simulink model "benchmark_ivan_PIANN"  (R2024b)
settings: Solver=FixedStepAuto  StartTime=0.0  StopTime=14  FixedStep=0.0001  RelTol=1e-5  AbsTol=1e-8  EnableMultiTasking=on
values from neighbouring files (symbols this model uses):
  b1 = csvread('./DAE_ANN/ANN/Biases/30_04_21/lstm_ann_pi_standard_fix_noSo4_rnn_1__100_16_b_3.csv')    [init_PI_ann.m]    (also in init_PI_ann_hier.m = csvread('./DAE_ANN/ANN/Biases/12_05_21/lstm_ann_pi_standard_; init_PI_ann_hier_v2.m = csvread('./DAE_ANN/ANN/Biases/12_05_21/lstm_ann_pi_standard_; init_PI_ann_lab.m = csvread('./DAE_ANN/ANN/Biases/12_05_21/lstm_ann_pi_standard_)
  b2 = csvread('./DAE_ANN/ANN/Biases/30_04_21/lstm_ann_pi_standard_fix_noSo4_rnn_1__100_16_b_3.csv')    [init_PI_ann.m]    (also in init_PI_ann_hier.m = csvread('./DAE_ANN/ANN/Biases/12_05_21/lstm_ann_pi_standard_; init_PI_ann_hier_v2.m = csvread('./DAE_ANN/ANN/Biases/12_05_21/lstm_ann_pi_standard_; init_PI_ann_lab.m = csvread('./DAE_ANN/ANN/Biases/12_05_21/lstm_ann_pi_standard_)
  b_last = csvread('./DAE_ANN/ANN/Biases/12_05_21/lstm_ann_pi_standard_fix_noSo4_last__100_1_b_2.csv')'    [init_PI_ann_hier.m]    (also in init_PI_ann_hier_v2.m; init_PI_ann_lab.m)
  b_out = csvread('./DAE_ANN/ANN/Biases/30_04_21/lstm_ann_pi_standard_fix_noSo4_final__100_16_b_3.csv')    [init_PI_ann.m]    (also in init_PI_ann_hier.m = csvread('./DAE_ANN/ANN/Biases/12_05_21/lstm_ann_pi_standard_; init_PI_ann_hier_v2.m = csvread('./DAE_ANN/ANN/Biases/12_05_21/lstm_ann_pi_standard_; init_PI_ann_lab.m = csvread('./DAE_ANN/ANN/Biases/12_05_21/lstm_ann_pi_standard_)
  ic_sw_Kla = 145*ones(n_sw,1)    [init_PI_ann.m]    (also in init_PI_ann_hier.m; init_PI_ann_hier_v2.m; init_PI_ann_lab.m)
  ic_sw_Snh4 = 6*ones(n_sw,1)    [init_PI_ann.m]    (also in init_PI_ann_hier.m; init_PI_ann_hier_v2.m; init_PI_ann_lab.m)
  ic_sw_Sno4 = 8*ones(n_sw,1)    [init_PI_ann.m]    (also in init_PI_ann_hier.m; init_PI_ann_hier_v2.m; init_PI_ann_lab.m)
  ic_sw_So4 = 3*ones(n_sw,1)    [init_PI_ann.m]    (also in init_PI_ann_hier.m; init_PI_ann_hier_v2.m; init_PI_ann_lab.m)
  ic_sw_So5 = 2*ones(n_sw,1)    [init_PI_ann.m]    (also in init_PI_ann_hier.m; init_PI_ann_hier_v2.m; init_PI_ann_lab.m)
  KLa5_max = 360    [sensorinit.m]
  max_Q4 = 100000    [sensorinit.m]
  max_SNH4 = 20    [sensorinit.m]
  max_SNO2 = 20    [sensorinit.m]
  max_SNO4 = 20    [sensorinit.m]
  max_SO4 = 10    [sensorinit.m]
  max_SO5 = 10    [sensorinit.m]    (also in setup_Prac5.m = 5)
  max_TSS4 = 10000    [sensorinit.m]
  mean_scaler_dir = csvread('./DAE_ANN/ANN/Scalers/30_04_21_lstm_ann_pi_standard_fix_noSo4/mean_scaler_lstm_ann_pi_standard_fix_noSo4.csv')    [init_PI_ann.m]    (also in init_PI_ann_hier.m = csvread('./DAE_ANN/ANN/Scalers/12_05_21_lstm_ann_pi_standard; init_PI_ann_hier_v2.m = csvread('./DAE_ANN/ANN/Scalers/12_05_21_lstm_ann_pi_standard; setup_Prac5.m = [(Q/k)^2, 1.9756, 0.0000, 0]')
  mean_scaler_dir_out = csvread('./DAE_ANN/ANN/Scalers/30_04_21_lstm_ann_pi_standard_fix_noSo4/mean_scaler_lstm_ann_pi_standard_fix_noSo4_out.csv')    [init_PI_ann.m]    (also in init_PI_ann_hier.m = csvread('./DAE_ANN/ANN/Scalers/12_05_21_lstm_ann_pi_standard; init_PI_ann_hier_v2.m = csvread('./DAE_ANN/ANN/Scalers/12_05_21_lstm_ann_pi_standard; setup_Prac5.m = 0)
  min_Q4 = 0    [sensorinit.m]
  min_SNH4 = 0    [sensorinit.m]
  min_SNO2 = 0    [sensorinit.m]
  min_SNO4 = 0    [sensorinit.m]
  min_SO5 = 0    [sensorinit.m]
  min_TSS4 = 0    [sensorinit.m]
  n_layers = 1    [init_PI_ann.m]    (also in init_PI_ann_hier.m; init_PI_ann_hier_v2.m; init_PI_ann_lab.m)
  n_sw = 16    [init_PI_ann.m]    (also in init_PI_ann_hier.m = 1; init_PI_ann_hier_v2.m = 1; init_PI_ann_lab.m = 1)
  n_sw_inverse = 16    [init_PI_ann.m]    (also in init_PI_ann_hier.m = 1; init_PI_ann_hier_v2.m = 1; init_PI_ann_lab.m = 1)
  noiseseed_Q4 = 1    [sensorinit.m]
  noiseseed_SNH4 = 2    [sensorinit.m]
  noiseseed_SNO2 = 2    [sensorinit.m]
  noiseseed_SNO4 = 2    [sensorinit.m]
  noiseseed_SO4 = 2    [sensorinit.m]
  noiseseed_SO5 = 1    [sensorinit.m]
  noiseseed_TSS4 = 1    [sensorinit.m]
  noisesource_Q4 = 1    [sensorinit.m]
  noisesource_SNH4 = 1    [sensorinit.m]
  noisesource_SNO2 = 1    [sensorinit.m]
  noisesource_SNO4 = 1    [sensorinit.m]
  noisesource_SO4 = 1    [sensorinit.m]
  noisesource_SO5 = 1    [sensorinit.m]
  noisesource_TSS4 = 1    [sensorinit.m]
  Qin0 = 18446    [states.mat]
  Qintr = 12141.8126939    [states.mat]
  Qintr_max = 5*Qin0    [sensorinit.m]
  Qintrawstate = 114243.527362    [states.mat]
  Qintrintstate = -116205.765277    [states.mat]
  SETTLERINIT = [12.5979803087 18.2981709885 29.6744598765 68.7829340492 352.293497132 353.981663079 351.499035887 351.323930185 355.679725774 6417.21684783 30 30 ... (80 elements, 1x80)]    [states.mat]
  Sno_mean = 1    [run_bsm1_PIANN_variable.m]
  SO5awstate = 469.399689831    [states.mat]
  SO5intstate = -450.70071346    [states.mat]
  SO5ref = 2    [run_bsm1_PIANN.m]    (also in run_bsm1_PIANN_variable.m)
  So_mean = 2    [run_bsm1_PIANN_variable.m]    (also in setup_Prac5.m = 0.2)
  std_Q4 = 0.025    [sensorinit.m]
  std_scaler_dir = csvread('./DAE_ANN/ANN/Scalers/30_04_21_lstm_ann_pi_standard_fix_noSo4/std_scaler_lstm_ann_pi_standard_fix_noSo4.csv')    [init_PI_ann.m]    (also in init_PI_ann_hier.m = csvread('./DAE_ANN/ANN/Scalers/12_05_21_lstm_ann_pi_standard; init_PI_ann_hier_v2.m = csvread('./DAE_ANN/ANN/Scalers/12_05_21_lstm_ann_pi_standard; setup_Prac5.m = [1, 0.7579, 0.05, 1]')
  std_scaler_dir_out = csvread('./DAE_ANN/ANN/Scalers/30_04_21_lstm_ann_pi_standard_fix_noSo4/std_scaler_lstm_ann_pi_standard_fix_noSo4_out.csv')    [init_PI_ann.m]    (also in init_PI_ann_hier.m = csvread('./DAE_ANN/ANN/Scalers/12_05_21_lstm_ann_pi_standard; init_PI_ann_hier_v2.m = csvread('./DAE_ANN/ANN/Scalers/12_05_21_lstm_ann_pi_standard; setup_Prac5.m = 1)
  std_SNH4 = 0.025    [sensorinit.m]
  std_SNO2 = 0.025    [sensorinit.m]
  std_SO4 = 0.025    [sensorinit.m]
  std_SO5 = 0.025    [sensorinit.m]
  std_TSS4 = 0.025    [sensorinit.m]
  T = 6.5201    [setup_Prac5.m]
  t_init = 7e-3    (= 0.007)    [run_bsm1.m]    (also in run_bsm1_PIANN_variable.m = 0.05)
  T_KLa5 = T90_KLa5/(24*60)/3.89    (= 0.000714081690945)    [sensorinit.m]
  T_Q4 = T90_Q4/(24*60)/3.89    (= 0.000178520422736)    [sensorinit.m]
  t_simulink = 1/96    (= 0.0104166666667)    [run_bsm1.m]    (also in run_bsm1_PIANN.m = -1; run_bsm1_PIANN_variable.m = 0; setup_Prac5.m = 0)
  T_SNH4 = T90_SNH4/(24*60)/11.7724    (= 0.000589891988417)    [sensorinit.m]
  T_SNO2 = T90_SNO2/(24*60)/11.7724    (= 0.000589891988417)    [sensorinit.m]
  T_SNO4 = T90_SNO4/(24*60)/11.7724    (= 0.000589891988417)    [sensorinit.m]
  T_SO5 = T90_SO5/(24*60)/3.89    (= 0.000178520422736)    [sensorinit.m]
  T_TSS4 = T90_TSS4/(24*60)/3.89    (= 0.000178520422736)    [sensorinit.m]
  t_zero_order = -1    [run_bsm1_PIANN.m]    (also in run_bsm1_PIANN_variable.m)
  u1 = csvread('./DAE_ANN/ANN/Weights/30_04_21/lstm_ann_pi_standard_fix_noSo4_rnn_1__100_16_U_3.csv')    [init_PI_ann.m]    (also in init_PI_ann_hier.m = csvread('./DAE_ANN/ANN/Weights/12_05_21/lstm_ann_pi_standard; init_PI_ann_hier_v2.m = csvread('./DAE_ANN/ANN/Weights/12_05_21/lstm_ann_pi_standard)
  u2 = csvread('./DAE_ANN/ANN/Weights/30_04_21/lstm_ann_pi_standard_fix_noSo4_rnn_1__100_16_U_3.csv')    [init_PI_ann.m]    (also in init_PI_ann_hier.m = csvread('./DAE_ANN/ANN/Weights/12_05_21/lstm_ann_pi_standard; init_PI_ann_hier_v2.m = csvread('./DAE_ANN/ANN/Weights/12_05_21/lstm_ann_pi_standard)
  useideal_KLa5 = 0    [run_bsm1.m]    (also in run_bsm1_PIANN.m = 1; run_bsm1_PIANN_variable.m = 1; sensorinit.m)
  useideal_Q4 = 1    [run_bsm1_PIANN.m]    (also in run_bsm1_PIANN_variable.m; sensorinit.m = 0)
  useideal_SNH4 = 0    [run_bsm1.m]    (also in run_bsm1_PIANN.m = 1; run_bsm1_PIANN_variable.m = 1; sensorinit.m)
  useideal_SNO2 = 1    [run_bsm1_PIANN.m]    (also in run_bsm1_PIANN_variable.m; sensorinit.m = 0)
  useideal_SNO4 = 0    [run_bsm1.m]    (also in run_bsm1_PIANN.m = 1; run_bsm1_PIANN_variable.m = 1; sensorinit.m)
  useideal_SO4 = 0    [run_bsm1.m]    (also in run_bsm1_PIANN.m = 1; run_bsm1_PIANN_variable.m = 1; sensorinit.m)
  useideal_SO5 = 0    [run_bsm1.m]    (also in run_bsm1_PIANN.m = 1; run_bsm1_PIANN_variable.m = 1; sensorinit.m)
  useideal_TSS4 = 1    [run_bsm1_PIANN.m]    (also in run_bsm1_PIANN_variable.m; sensorinit.m = 0)
  usenoise_Q4 = 0    [run_bsm1_PIANN.m]    (also in run_bsm1_PIANN_variable.m; sensorinit.m = 1)
  usenoise_SNH4 = 1    [run_bsm1.m]    (also in run_bsm1_PIANN.m = 0; run_bsm1_PIANN_variable.m = 0; sensorinit.m)
  usenoise_SNO2 = 0    [run_bsm1_PIANN.m]    (also in run_bsm1_PIANN_variable.m; sensorinit.m = 1)
  usenoise_SNO4 = 1    [run_bsm1.m]    (also in run_bsm1_PIANN.m = 0; run_bsm1_PIANN_variable.m = 0; sensorinit.m)
  usenoise_SO4 = 1    [run_bsm1.m]    (also in run_bsm1_PIANN.m = 0; run_bsm1_PIANN_variable.m = 0; sensorinit.m)
  usenoise_SO5 = 1    [run_bsm1.m]    (also in run_bsm1_PIANN.m = 0; run_bsm1_PIANN_variable.m = 0; sensorinit.m)
  usenoise_TSS4 = 0    [run_bsm1_PIANN.m]    (also in run_bsm1_PIANN_variable.m; sensorinit.m = 1)
  w1 = csvread('./DAE_ANN/ANN/Weights/30_04_21/lstm_ann_pi_standard_fix_noSo4_rnn_1__100_16_W_3.csv')    [init_PI_ann.m]    (also in init_PI_ann_hier.m = csvread('./DAE_ANN/ANN/Weights/12_05_21/lstm_ann_pi_standard; init_PI_ann_hier_v2.m = csvread('./DAE_ANN/ANN/Weights/12_05_21/lstm_ann_pi_standard; init_PI_ann_lab.m = csvread('./DAE_ANN/ANN/Weights/12_05_21/lstm_ann_pi_standard)
  w2 = csvread('./DAE_ANN/ANN/Weights/30_04_21/lstm_ann_pi_standard_fix_noSo4_rnn_1__100_16_W_3.csv')    [init_PI_ann.m]    (also in init_PI_ann_hier.m = csvread('./DAE_ANN/ANN/Weights/12_05_21/lstm_ann_pi_standard; init_PI_ann_hier_v2.m = csvread('./DAE_ANN/ANN/Weights/12_05_21/lstm_ann_pi_standard; init_PI_ann_lab.m = csvread('./DAE_ANN/ANN/Weights/12_05_21/lstm_ann_pi_standard)
  w_last = csvread('./DAE_ANN/ANN/Weights/12_05_21/lstm_ann_pi_standard_fix_noSo4_last__100_1_W_2.csv')    [init_PI_ann_hier.m]    (also in init_PI_ann_hier_v2.m; init_PI_ann_lab.m)
  w_out = csvread('./DAE_ANN/ANN/Weights/30_04_21/lstm_ann_pi_standard_fix_noSo4_final__100_16_W_3.csv')    [init_PI_ann.m]    (also in init_PI_ann_hier.m = csvread('./DAE_ANN/ANN/Weights/12_05_21/lstm_ann_pi_standard; init_PI_ann_hier_v2.m = csvread('./DAE_ANN/ANN/Weights/12_05_21/lstm_ann_pi_standard; init_PI_ann_lab.m = csvread('./DAE_ANN/ANN/Weights/12_05_21/lstm_ann_pi_standard)
  XINIT1 = [30 3.2250440682 1132.84750814 98.0848162551 2520.32093658 147.34360098 454.498440184 0.006943357113 3.54207658602 12.0720627837 1.35151294762 6.05742445882 ... (15 elements, 1x15)]    [states.mat]
  XINIT2 = [30 1.63865407136 1124.24951453 88.653599068 2501.35826654 146.001740625 452.094465666 5.17099136584e-05 1.14245691502 13.0383387996 0.796493225193 5.70045637375 ... (15 elements, 1x15)]    [states.mat]
  XINIT3 = [30 1.20592174915 1120.58961418 67.1871738861 2499.94635325 146.547839977 452.007772249 1.74081325353 6.26492922945 8.40116301472 0.827753486834 4.51387309735 ... (15 elements, 1x15)]    [states.mat]
  XINIT4 = [30 0.96656120797 1121.66055561 52.7833355811 2504.32671079 147.644975737 453.890499756 2.40137566232 11.073804945 3.99279026202 0.746788866766 3.70339113264 ... (15 elements, 1x15)]    [states.mat]
  XINIT5 = [30 0.803395489358 1124.12455116 43.2595495328 2508.23031357 148.499403125 456.322790044 2.11978031988 14.1356901459 1.15379834533 0.659650038761 3.15951382084 ... (15 elements, 1x15)]    [states.mat]
  XINITDELAY = [1466770.04249 1266021.87556 55799754.9774 5815431.95778 123179806.598 7263098.80912 22318785.5012 62039.7687555 416609.519268 588047.303413 143684.636473 343270.852984 ... (15 elements, 1x15)]    [states.mat]
undefined symbols (not defined in the file or in its folder): b_bottle, b_decoder_1, b_decoder_2, b_encoder_1, b_encoder_2, b_final, b_out_dae, carb1, carb2, carb3, carb4, carb5, DIM, Kfeedforward, KLa1, KLa2, KLa3, KLa4, KLa5offset, KQintr, KSO5, LAYER, magnitude, mean_scaler_dae, mean_scaler_dae_out, MODELTYPE, PAR1, PAR2, PAR3, PAR4, PAR5, Qffref, Qintroffset, QintrT, SETTLERPAR, SNO2ref, SOSAT1, SOSAT2, SOSAT3, SOSAT4, SOSAT5, std_scaler_dae, std_scaler_dae_out, TiQintr, TiSO5, TtQintr, TtSO5, u_decoder_1, u_decoder_2, u_encoder_1, u_encoder_2, useantiwindupQintr, useantiwindupSO5, VOL1, VOL2, VOL3, VOL4, VOL5, w_bottle, w_decoder_1 ... (+5)
libraries: dspindex x33
(part 3 of 4)

== system benchmark_ivan_PIANN/SO5_control_paper/Filter_Prediction/DAE_lstm/Data Preprocessing Direct1 ==
  y_n : Inport
  Denormalization Values : MATLAB Function  TreatAsAtomicUnit=on
  Out1 : Outport  VectorParamsAs1DForOutWhenUnconnected=off
  wires:
  Denormalization Values/1(data_dir) -> Out1/1
  y_n/1 -> Denormalization Values/1(data_input)

== system benchmark_ivan_PIANN/SO5_control_paper/Filter_Prediction/DAE_lstm/Sliding Window ==
  So4 : Inport
  Sno4 : Inport  Port=2
  Snh4 : Inport  Port=3
  So5 : Inport  Port=4
  Matrix Concatenate : Concatenate  NumInputs=4  Mode=Multidimensional array  ConcatenateDimension=2
  Sliding Window1 : Subsystem  Commented=on
  Sliding Window2 : Subsystem
  Sliding Window3 : Subsystem
  Sliding Window4 : Subsystem
  Sliding Window6 : Subsystem
  Out1 : Outport  VectorParamsAs1DForOutWhenUnconnected=off
  wires:
  Sliding Window6/1(Out) -> Matrix Concatenate/1
  Sliding Window2/1(Out) -> Matrix Concatenate/2
  Matrix Concatenate/1 -> Out1/1
  Sliding Window3/1(Out) -> Matrix Concatenate/3
  So4/1 -> Sliding Window6/1(In)
  Sno4/1 -> Sliding Window2/1(In)
  Snh4/1 -> Sliding Window3/1(In)
  So5/1 -> Sliding Window4/1(In)
  Sliding Window4/1(Out) -> Matrix Concatenate/4

== system benchmark_ivan_PIANN/SO5_control_paper/Filter_Prediction/Direct Prediction LSTM4/Data Preprocesing Direct ==
  u_n : Inport
  Math Function : Math  Operator=transpose  SignedPower=on
  Normalization Values : MATLAB Function  TreatAsAtomicUnit=on
  Reshape : Reshape  OutputDimensionality=Row vector (2-D)
  Out1 : Outport  VectorParamsAs1DForOutWhenUnconnected=off
  wires:
  Reshape/1 -> Out1/1
  Normalization Values/1(data_norm) -> Math Function/1
  Math Function/1 -> Reshape/1
  u_n/1 -> Normalization Values/1(data_input)

== system benchmark_ivan_PIANN/SO5_control_paper/Filter_Prediction/Direct Prediction LSTM4/Data Preprocessing Direct1 ==
  y_n : Inport
  Denormalization Values : MATLAB Function  TreatAsAtomicUnit=on
  Out1 : Outport  VectorParamsAs1DForOutWhenUnconnected=off
  wires:
  y_n/1 -> Denormalization Values/1(data_input)
  Denormalization Values/1(data_dir) -> Out1/1

== system benchmark_ivan_PIANN/SO5_control_paper/Filter_Prediction/Direct Prediction LSTM4/Direct ANN ==
  x_norm : Inport
  Predict RNN Ntot Keras : MATLAB Function  TreatAsAtomicUnit=on
  y_n : Outport  VectorParamsAs1DForOutWhenUnconnected=off
  wires:
  Predict RNN Ntot Keras/1(prediction) -> y_n/1
  x_norm/1 -> Predict RNN Ntot Keras/1(data_in)

== system benchmark_ivan_PIANN/SO5_control_paper/Filter_Prediction/Direct Prediction LSTM4/Sliding Window 1 ==
  data1 : Inport
  ref : Inport  Port=2
  Matrix Concatenate : Concatenate  NumInputs=5  Mode=Multidimensional array  ConcatenateDimension=2
  Reshape{1,3..5} (4 alike) : Reshape
  Select_Snh1 : Selector  NumberOfDimensions=2  InputPortWidth=4  IndexOptions=Index vector (dialog),Index vector (dialog)  Indices=1,[4:4:64]  OutputSizes=1,1
  Select_Snh2 : Selector  NumberOfDimensions=2  InputPortWidth=4  IndexOptions=Index vector (dialog),Index vector (dialog)  Indices=1,[3:4:64]  OutputSizes=1,1
  Select_Sno1 : Selector  NumberOfDimensions=2  InputPortWidth=4  IndexOptions=Index vector (dialog),Index vector (dialog)  Indices=1,[2:4:64]  OutputSizes=1,1
  Select_So1 : Selector  NumberOfDimensions=2  InputPortWidth=4  IndexOptions=Index vector (dialog),Index vector (dialog)  Indices=1,[1:4:64]  OutputSizes=1,1
  Sliding Window Buffer : Subsystem
  Sliding Window2 : Subsystem  Commented=on
  Out1 : Outport  VectorParamsAs1DForOutWhenUnconnected=off
  wires:
  Matrix Concatenate/1 -> Out1/1
  data1/1 -> Select_Snh1/1, Select_Snh2/1, Select_Sno1/1, Select_So1/1
  ref/1 -> Sliding Window Buffer/1(In1)
  Select_Snh2/1 -> Reshape5/1
  Select_Sno1/1 -> Reshape4/1
  Select_So1/1 -> Reshape3/1
  Reshape3/1 -> Matrix Concatenate/1
  Reshape4/1 -> Matrix Concatenate/2
  Reshape5/1 -> Matrix Concatenate/3
  Sliding Window Buffer/1(Out1) -> Matrix Concatenate/5
  Reshape1/1 -> Matrix Concatenate/4
  Select_Snh1/1 -> Reshape1/1

== system benchmark_ivan_PIANN/SO5_control_paper/Filter_Prediction/Direct Prediction LSTM4/Sliding Window 48  ==
  data1 : Inport
  ref : Inport  Port=2
  Matrix Concatenate : Concatenate  NumInputs=6  Mode=Multidimensional array  ConcatenateDimension=2
  Reshape{1..5} (5 alike) : Reshape
  Select_Q4 : Selector  NumberOfDimensions=2  InputPortWidth=4  IndexOptions=Index vector (dialog),Index vector (dialog)  Indices=1,[3:5:80]  OutputSizes=1,1
  Select_Snh4 : Selector  NumberOfDimensions=2  InputPortWidth=4  IndexOptions=Index vector (dialog),Index vector (dialog)  Indices=1,[1:5:80]  OutputSizes=1,1
  Select_So5 : Selector  NumberOfDimensions=2  InputPortWidth=4  IndexOptions=Index vector (dialog),Index vector (dialog)  Indices=1,[4:5:80]  OutputSizes=1,1
  Select_TSS4 : Selector  NumberOfDimensions=2  InputPortWidth=4  IndexOptions=Index vector (dialog),Index vector (dialog)  Indices=1,[2:5:80]  OutputSizes=1,1
  Select_TSSin : Selector  NumberOfDimensions=2  InputPortWidth=4  IndexOptions=Index vector (dialog),Index vector (dialog)  Indices=1,[5:5:80]  OutputSizes=1,1
  Sliding Window1 : Subsystem  Commented=on
  Sliding Window2 : Subsystem
  Out1 : Outport  VectorParamsAs1DForOutWhenUnconnected=off
  wires:
  Matrix Concatenate/1 -> Out1/1
  ref/1 -> Sliding Window2/1(In)
  Select_Q4/1 -> Reshape5/1
  Reshape3/1 -> Matrix Concatenate/1
  Select_Snh4/1 -> Reshape3/1
  Reshape5/1 -> Matrix Concatenate/3
  Select_TSS4/1 -> Reshape4/1
  Reshape4/1 -> Matrix Concatenate/2
  Select_So5/1 -> Reshape1/1
  data1/1 -> Select_Snh4/1, Select_TSS4/1, Select_Q4/1, Select_TSSin/1, Select_So5/1
  Select_TSSin/1 -> Reshape2/1
  Sliding Window2/1(Out) -> Matrix Concatenate/4
  Reshape1/1 -> Matrix Concatenate/5
  Reshape2/1 -> Matrix Concatenate/6

== system benchmark_ivan_PIANN/SO5_control_paper/Filter_Prediction/Direct Prediction LSTM4/Sliding Window 64 ==
  data1 : Inport
  ref : Inport  Port=2
  Matrix Concatenate : Concatenate  NumInputs=4  Mode=Multidimensional array  ConcatenateDimension=2
  Reshape3 : Reshape
  Reshape4 : Reshape
  Reshape5 : Reshape
  Select_Snh2 : Selector  NumberOfDimensions=2  InputPortWidth=4  IndexOptions=Index vector (dialog),Index vector (dialog)  Indices=1,[3:4:64]  OutputSizes=1,1
  Select_Sno1 : Selector  NumberOfDimensions=2  InputPortWidth=4  IndexOptions=Index vector (dialog),Index vector (dialog)  Indices=1,[2:4:64]  OutputSizes=1,1
  Select_So1 : Selector  NumberOfDimensions=2  InputPortWidth=4  IndexOptions=Index vector (dialog),Index vector (dialog)  Indices=1,[1:4:64]  OutputSizes=1,1
  Sliding Window1 : Subsystem  Commented=on
  Sliding Window2 : Subsystem
  Out1 : Outport  VectorParamsAs1DForOutWhenUnconnected=off
  wires:
  Matrix Concatenate/1 -> Out1/1
  ref/1 -> Sliding Window2/1(In)
  Sliding Window2/1(Out) -> Matrix Concatenate/4
  Select_Snh2/1 -> Reshape5/1
  Reshape3/1 -> Matrix Concatenate/1
  Select_So1/1 -> Reshape3/1
  Reshape5/1 -> Matrix Concatenate/3
  Select_Sno1/1 -> Reshape4/1
  data1/1 -> Select_So1/1, Select_Snh2/1, Select_Sno1/1
  Reshape4/1 -> Matrix Concatenate/2

== system benchmark_ivan_PIANN/SO5_control_paper/Filter_Prediction/Direct Prediction LSTM4/Sliding Window 64 with So5 ==
  data1 : Inport
  ref : Inport  Port=2
  Matrix Concatenate : Concatenate  NumInputs=5  Mode=Multidimensional array  ConcatenateDimension=2
  Reshape{1,3..5} (4 alike) : Reshape
  Select_Snh1 : Selector  NumberOfDimensions=2  InputPortWidth=4  IndexOptions=Index vector (dialog),Index vector (dialog)  Indices=1,[4:4:64]  OutputSizes=1,1
  Select_Snh2 : Selector  NumberOfDimensions=2  InputPortWidth=4  IndexOptions=Index vector (dialog),Index vector (dialog)  Indices=1,[3:4:64]  OutputSizes=1,1
  Select_Sno1 : Selector  NumberOfDimensions=2  InputPortWidth=4  IndexOptions=Index vector (dialog),Index vector (dialog)  Indices=1,[2:4:64]  OutputSizes=1,1
  Select_So1 : Selector  NumberOfDimensions=2  InputPortWidth=4  IndexOptions=Index vector (dialog),Index vector (dialog)  Indices=1,[1:4:64]  OutputSizes=1,1
  Sliding Window1 : Subsystem  Commented=on
  Sliding Window2 : Subsystem
  Out1 : Outport  VectorParamsAs1DForOutWhenUnconnected=off
  wires:
  Matrix Concatenate/1 -> Out1/1
  ref/1 -> Sliding Window2/1(In)
  Select_Snh2/1 -> Reshape5/1
  Reshape3/1 -> Matrix Concatenate/1
  Select_So1/1 -> Reshape3/1
  Reshape5/1 -> Matrix Concatenate/3
  Select_Sno1/1 -> Reshape4/1
  Reshape4/1 -> Matrix Concatenate/2
  data1/1 -> Select_So1/1, Select_Snh1/1, Select_Snh2/1, Select_Sno1/1
  Select_Snh1/1 -> Reshape1/1
  Sliding Window2/1(Out) -> Matrix Concatenate/4
  Reshape1/1 -> Matrix Concatenate/5

== system benchmark_ivan_PIANN/SO5_control_paper/Filter_Prediction/Inverse Data/ Q4_sensor_(A) ==
  note: SENSOR CLASS: A
  u : Inport
  Constant : Constant  Value=usenoise_Q4
  Constant1 : Constant  Value=noisesource_Q4
  Constant2 : Constant  Value=useideal_Q4
  From Workspace : FromWorkspace  VariableName=NOISEDATA_Q4  ZeroCross=off
  Gain : Gain  Gain=max_Q4*std_Q4  SaturateOnIntegerOverflow=on  OutDataTypeStr=Inherit: Same as input  ParamDataTypeStr=Inherit: Same as input
  Mux : Mux  Inputs=6
  Product : Product  InputSameDT=on  SaturateOnIntegerOverflow=on  OutDataTypeStr=Inherit: Same as first input
  Random Number : RandomNumber  Seed=noiseseed_Q4  SampleTime=1/1440
  Saturation : Saturate  UpperLimit=max_Q4  LowerLimit=min_Q4
  Select_DO : Selector  InputPortWidth=15  IndexOptions=Index vector (dialog)  Indices=[15]  OutputSizes=1
  Sum : Sum  Inputs=|++  InputSameDT=on  SaturateOnIntegerOverflow=on  OutDataTypeStr=Inherit: Same as first input
  Switch : Switch  Threshold=0.5  SaturateOnIntegerOverflow=off  InputSameDT=off
  Switch1 : Switch  Threshold=0.5  SaturateOnIntegerOverflow=off  InputSameDT=off
  To Workspace : ToWorkspace  VariableName=Q4sensor_aux  SampleTime=-1
  second order Laplace : TransferFcn  Denominator=[ T_Q4*T_Q4, 2*T_Q4, 1]
  y : Outport  VectorParamsAs1DForOutWhenUnconnected=off
  wires:
  Mux/1 -> To Workspace/1
  Constant2/1 -> Switch1/2
  Switch1/1 -> Mux/6, y/1
  Saturation/1 -> Switch1/3
  Random Number/1 -> Switch/3
  Constant1/1 -> Switch/2
  From Workspace/1 -> Switch/1
  Constant/1 -> Product/1
  Switch/1 -> Gain/1
  Gain/1 -> Product/2
  Select_DO/1 -> Mux/1, Switch1/1, second order Laplace/1
  u/1 -> Select_DO/1
  Product/1 -> Mux/4, Sum/2
  second order Laplace/1 -> Mux/3, Mux/2, Sum/1
  Sum/1 -> Mux/5, Saturation/1

== system benchmark_ivan_PIANN/SO5_control_paper/Filter_Prediction/Inverse Data/SNH4_sensor_(B0) ==
  note: SENSOR CLASS: B0
  u : Inport
  Constant : Constant  Value=usenoise_SNH4
  Constant1 : Constant  Value=noisesource_SNH4
  Constant2 : Constant  Value=useideal_SNH4
  From Workspace : FromWorkspace  VariableName=NOISEDATA_SNH4  ZeroCross=off
  Gain : Gain  Gain=max_SNH4*std_SNH4  SaturateOnIntegerOverflow=on  OutDataTypeStr=Inherit: Same as input  ParamDataTypeStr=Inherit: Same as input
  Mux : Mux  Inputs=6
  Product : Product  InputSameDT=on  SaturateOnIntegerOverflow=on  OutDataTypeStr=Inherit: Same as first input
  Random Number : RandomNumber  Seed=noiseseed_SNH4  SampleTime=1/1440
  Saturation : Saturate  UpperLimit=max_SNH4  LowerLimit=min_SNH4
  Select_SNO : Selector  InputPortWidth=15  IndexOptions=Index vector (dialog)  Indices=[10]  OutputSizes=1
  Sum : Sum  Inputs=|++  InputSameDT=on  SaturateOnIntegerOverflow=on  OutDataTypeStr=Inherit: Same as first input
  Switch : Switch  Threshold=0.5  SaturateOnIntegerOverflow=off  InputSameDT=off
  Switch1 : Switch  Threshold=0.5  SaturateOnIntegerOverflow=off  InputSameDT=off
  To Workspace : ToWorkspace  VariableName=SNH4sensor  SampleTime=-1
  eight order Laplace : TransferFcn  Denominator=[ T_SNH4*T_SNH4*T_SNH4*T_SNH4*T_SNH4*T_SNH4*T_SNH4*T_SNH4, 8*T_SNH4*T_SNH4*T_SNH4*T_SNH4*T_SNH4*T_SNH4*T_SNH4, 28*T_SNH4*T_SNH4*T_SNH4*T_SNH4*T_SNH4*T_SNH4, 56*T_SNH4*T_SNH4*T_SNH4*T_SNH4*T_SNH4, 70*T_SNH4*T_SNH4*T_SNH4*T_SNH4, 56*T_SNH4*T_SNH4*T_SNH4, 28*T_SNH4*T_SNH4, 8* T_SNH4, 1]
  y : Outport  VectorParamsAs1DForOutWhenUnconnected=off
  wires:
  Mux/1 -> To Workspace/1
  Constant2/1 -> Switch1/2
  Switch1/1 -> Mux/6, y/1
  Saturation/1 -> Switch1/3
  Random Number/1 -> Switch/3
  Constant1/1 -> Switch/2
  From Workspace/1 -> Switch/1
  Constant/1 -> Product/1
  Switch/1 -> Gain/1
  Gain/1 -> Product/2
  Select_SNO/1 -> Mux/1, Switch1/1, eight order Laplace/1
  u/1 -> Select_SNO/1
  Product/1 -> Mux/4, Sum/2
  eight order Laplace/1 -> Mux/3, Mux/2, Sum/1
  Sum/1 -> Mux/5, Saturation/1

== system benchmark_ivan_PIANN/SO5_control_paper/Filter_Prediction/Inverse Data/TSS4_sensor_(A) ==
  note: SENSOR CLASS: A
  u : Inport
  Constant : Constant  Value=usenoise_TSS4
  Constant1 : Constant  Value=noisesource_TSS4
  Constant2 : Constant  Value=useideal_TSS4
  From Workspace : FromWorkspace  VariableName=NOISEDATA_TSS4  ZeroCross=off
  Gain : Gain  Gain=max_TSS4*std_TSS4  SaturateOnIntegerOverflow=on  OutDataTypeStr=Inherit: Same as input  ParamDataTypeStr=Inherit: Same as input
  Mux : Mux  Inputs=6
  Product : Product  InputSameDT=on  SaturateOnIntegerOverflow=on  OutDataTypeStr=Inherit: Same as first input
  Random Number : RandomNumber  Seed=noiseseed_TSS4  SampleTime=1/1440
  Saturation : Saturate  UpperLimit=max_TSS4  LowerLimit=min_TSS4
  Select_DO : Selector  InputPortWidth=15  IndexOptions=Index vector (dialog)  Indices=[14]  OutputSizes=1
  Sum : Sum  Inputs=|++  InputSameDT=on  SaturateOnIntegerOverflow=on  OutDataTypeStr=Inherit: Same as first input
  Switch : Switch  Threshold=0.5  SaturateOnIntegerOverflow=off  InputSameDT=off
  Switch1 : Switch  Threshold=0.5  SaturateOnIntegerOverflow=off  InputSameDT=off
  To Workspace : ToWorkspace  VariableName=TSS4sensor_aux  SampleTime=-1
  second order Laplace : TransferFcn  Denominator=[ T_TSS4*T_TSS4, 2*T_TSS4, 1]
  y : Outport  VectorParamsAs1DForOutWhenUnconnected=off
  wires:
  Mux/1 -> To Workspace/1
  Constant2/1 -> Switch1/2
  Switch1/1 -> Mux/6, y/1
  Saturation/1 -> Switch1/3
  Random Number/1 -> Switch/3
  Constant1/1 -> Switch/2
  From Workspace/1 -> Switch/1
  Constant/1 -> Product/1
  Switch/1 -> Gain/1
  Gain/1 -> Product/2
  Select_DO/1 -> Mux/1, Switch1/1, second order Laplace/1
  u/1 -> Select_DO/1
  Product/1 -> Mux/4, Sum/2
  second order Laplace/1 -> Mux/3, Mux/2, Sum/1
  Sum/1 -> Mux/5, Saturation/1

== system benchmark_ivan_PIANN/SO5_control_paper/Filter_Prediction/DAE_MLP1/Sliding Window/Sliding Window3 ==
  In : Inport
  Delay1 : Delay  DelayLength=1  InitialCondition=0  SampleTime=t_simulink
  Flip : DSPFlip
  IC : InitialCondition  Value=ic_sw_Snh4
  Mux : Mux  Inputs=2
  To Workspace5 : ToWorkspace  VariableName=sw_Snh4  SampleTime=1/96
  Variable Selector : dspindex/Variable Selector  NumInputs=1  rowsOrCols=Rows  IdxMode=Fixed  Elements=1:(n_sw_inverse-1)  ZerOneIdxMode=One-based  errmode=Clip Index  FillMode=on  FillValues=0
  Out : Outport  VectorParamsAs1DForOutWhenUnconnected=off
  wires:
  IC/1 -> Variable Selector/1
  Delay1/1 -> IC/1
  In/1 -> Mux/1
  Variable Selector/1 -> Mux/2
  Flip/1 -> To Workspace5/1, Out/1
  Mux/1 -> Delay1/1, Flip/1

== system benchmark_ivan_PIANN/SO5_control_paper/Filter_Prediction/DAE_MLP1/Sliding Window/Sliding Window4 ==
  In : Inport
  Delay1 : Delay  DelayLength=1  InitialCondition=0  SampleTime=t_simulink
  Flip : DSPFlip
  IC : InitialCondition  Value=ic_sw_Sno4
  Mux : Mux  Inputs=2
  To Workspace5 : ToWorkspace  VariableName=sw_Sno4  SampleTime=1/96
  Variable Selector : dspindex/Variable Selector  NumInputs=1  rowsOrCols=Rows  IdxMode=Fixed  Elements=1:(n_sw_inverse-1)  ZerOneIdxMode=One-based  errmode=Clip Index  FillMode=on  FillValues=0
  Out : Outport  VectorParamsAs1DForOutWhenUnconnected=off
  wires:
  IC/1 -> Variable Selector/1
  Delay1/1 -> IC/1
  In/1 -> Mux/1
  Variable Selector/1 -> Mux/2
  Flip/1 -> To Workspace5/1, Out/1
  Mux/1 -> Delay1/1, Flip/1

== system benchmark_ivan_PIANN/SO5_control_paper/Filter_Prediction/DAE_MLP1/Sliding Window/Sliding Window6 ==
  In : Inport
  Delay1 : Delay  DelayLength=1  InitialCondition=0  SampleTime=t_simulink
  Flip : DSPFlip
  IC : InitialCondition  Value=ic_sw_So4
  Mux : Mux  Inputs=2
  To Workspace5 : ToWorkspace  VariableName=sw_So4  SampleTime=1/96
  Variable Selector : dspindex/Variable Selector  NumInputs=1  rowsOrCols=Rows  IdxMode=Fixed  Elements=1:(n_sw_inverse-1)  ZerOneIdxMode=One-based  errmode=Clip Index  FillMode=on  FillValues=0
  Out : Outport  VectorParamsAs1DForOutWhenUnconnected=off
  wires:
  IC/1 -> Variable Selector/1
  Delay1/1 -> IC/1
  In/1 -> Mux/1
  Variable Selector/1 -> Mux/2
  Flip/1 -> To Workspace5/1, Out/1
  Mux/1 -> Delay1/1, Flip/1

== system benchmark_ivan_PIANN/SO5_control_paper/Filter_Prediction/DAE_MLP2/Sliding Window/Sliding Window1 ==
  In : Inport
  Delay1 : Delay  DelayLength=1  InitialCondition=0  SampleTime=t_simulink
  Flip : DSPFlip
  IC : InitialCondition  Value=ic_sw_So5
  Mux : Mux  Inputs=2
  To Workspace5 : ToWorkspace  VariableName=sw_So5  SampleTime=1/96
  Variable Selector : dspindex/Variable Selector  NumInputs=1  rowsOrCols=Rows  IdxMode=Fixed  Elements=1:(n_sw_inverse-1)  ZerOneIdxMode=One-based  errmode=Clip Index  FillMode=on  FillValues=0
  Out : Outport  VectorParamsAs1DForOutWhenUnconnected=off
  wires:
  IC/1 -> Variable Selector/1
  Delay1/1 -> IC/1
  In/1 -> Mux/1
  Variable Selector/1 -> Mux/2
  Flip/1 -> To Workspace5/1, Out/1
  Mux/1 -> Delay1/1, Flip/1

== system benchmark_ivan_PIANN/SO5_control_paper/Filter_Prediction/DAE_MLP2/Sliding Window/Sliding Window2 ==
  In : Inport
  Delay1 : Delay  DelayLength=1  InitialCondition=0  SampleTime=t_simulink
  Flip : DSPFlip
  IC : InitialCondition  Value=ic_sw_Snh4
  Mux : Mux  Inputs=2
  To Workspace5 : ToWorkspace  VariableName=sw_Snh4  SampleTime=1/96
  Variable Selector : dspindex/Variable Selector  NumInputs=1  rowsOrCols=Rows  IdxMode=Fixed  Elements=1:(n_sw_inverse-1)  ZerOneIdxMode=One-based  errmode=Clip Index  FillMode=on  FillValues=0
  Out : Outport  VectorParamsAs1DForOutWhenUnconnected=off
  wires:
  IC/1 -> Variable Selector/1
  Delay1/1 -> IC/1
  In/1 -> Mux/1
  Variable Selector/1 -> Mux/2
  Flip/1 -> To Workspace5/1, Out/1
  Mux/1 -> Delay1/1, Flip/1

== system benchmark_ivan_PIANN/SO5_control_paper/Filter_Prediction/DAE_MLP2/Sliding Window/Sliding Window5 ==
  In : Inport
  Delay1 : Delay  DelayLength=1  InitialCondition=0  SampleTime=t_simulink
  Flip : DSPFlip
  IC : InitialCondition  Value=ic_sw_Sno4
  Mux : Mux  Inputs=2
  To Workspace5 : ToWorkspace  VariableName=sw_Sno4  SampleTime=1/96
  Variable Selector : dspindex/Variable Selector  NumInputs=1  rowsOrCols=Rows  IdxMode=Fixed  Elements=1:(n_sw_inverse-1)  ZerOneIdxMode=One-based  errmode=Clip Index  FillMode=on  FillValues=0
  Out : Outport  VectorParamsAs1DForOutWhenUnconnected=off
  wires:
  IC/1 -> Variable Selector/1
  Delay1/1 -> IC/1
  In/1 -> Mux/1
  Variable Selector/1 -> Mux/2
  Flip/1 -> To Workspace5/1, Out/1
  Mux/1 -> Delay1/1, Flip/1

== system benchmark_ivan_PIANN/SO5_control_paper/Filter_Prediction/DAE_MLP2/Sliding Window/Sliding Window7 ==
  In : Inport
  Delay1 : Delay  DelayLength=1  InitialCondition=0  SampleTime=t_simulink
  Flip : DSPFlip
  IC : InitialCondition  Value=ic_sw_So4
  Mux : Mux  Inputs=2
  To Workspace5 : ToWorkspace  VariableName=sw_So4  SampleTime=1/96
  Variable Selector : dspindex/Variable Selector  NumInputs=1  rowsOrCols=Rows  IdxMode=Fixed  Elements=1:(n_sw_inverse-1)  ZerOneIdxMode=One-based  errmode=Clip Index  FillMode=on  FillValues=0
  Out : Outport  VectorParamsAs1DForOutWhenUnconnected=off
  wires:
  IC/1 -> Variable Selector/1
  Delay1/1 -> IC/1
  In/1 -> Mux/1
  Variable Selector/1 -> Mux/2
  Flip/1 -> To Workspace5/1, Out/1
  Mux/1 -> Delay1/1, Flip/1

== system benchmark_ivan_PIANN/SO5_control_paper/Filter_Prediction/DAE_MLP3/Sliding Window/Sliding Window Buffer Snh4 ==
  In1 : Inport
  Buffer1 : Buffer  N=n_sw  V=n_sw-1  ic=6
  Reshape : Reshape
  To Workspace5 : ToWorkspace  VariableName=sw_Snh4  SampleTime=-1
  Zero-Order Hold : ZeroOrderHold  SampleTime=-1
  Out1 : Outport
  wires:
  Buffer1/1 -> Reshape/1
  Reshape/1 -> To Workspace5/1, Out1/1
  In1/1 -> Zero-Order Hold/1
  Zero-Order Hold/1 -> Buffer1/1

== system benchmark_ivan_PIANN/SO5_control_paper/Filter_Prediction/DAE_MLP3/Sliding Window/Sliding Window Buffer Sno4 ==
  In1 : Inport
  Buffer1 : Buffer  N=n_sw  V=n_sw-1  ic=92230
  Reshape : Reshape
  To Workspace5 : ToWorkspace  VariableName=sw_Sno4  SampleTime=-1
  Zero-Order Hold : ZeroOrderHold  SampleTime=-1
  Out1 : Outport
  wires:
  Buffer1/1 -> Reshape/1
  Reshape/1 -> To Workspace5/1, Out1/1
  In1/1 -> Zero-Order Hold/1
  Zero-Order Hold/1 -> Buffer1/1

== system benchmark_ivan_PIANN/SO5_control_paper/Filter_Prediction/DAE_MLP3/Sliding Window/Sliding Window Buffer So4 ==
  In1 : Inport
  Buffer1 : Buffer  N=n_sw  V=n_sw-1  ic=3220.1
  Reshape : Reshape
  To Workspace5 : ToWorkspace  VariableName=sw_TSS4  SampleTime=-1
  Zero-Order Hold : ZeroOrderHold  SampleTime=-1
  Out1 : Outport
  wires:
  Buffer1/1 -> Reshape/1
  Reshape/1 -> To Workspace5/1, Out1/1
  In1/1 -> Zero-Order Hold/1
  Zero-Order Hold/1 -> Buffer1/1

== system benchmark_ivan_PIANN/SO5_control_paper/Filter_Prediction/DAE_MLP3/Sliding Window/Sliding Window Buffer So5 ==
  In1 : Inport
  Buffer1 : Buffer  N=n_sw  V=n_sw-1  ic=2
  Reshape : Reshape
  To Workspace5 : ToWorkspace  VariableName=sw_So5  SampleTime=-1
  Zero-Order Hold : ZeroOrderHold  SampleTime=-1
  Out1 : Outport
  wires:
  Buffer1/1 -> Reshape/1
  Reshape/1 -> To Workspace5/1, Out1/1
  In1/1 -> Zero-Order Hold/1
  Zero-Order Hold/1 -> Buffer1/1

== system benchmark_ivan_PIANN/SO5_control_paper/Filter_Prediction/DAE_MLP3/Sliding Window/Sliding Window1 ==
  In : Inport
  Delay1 : Delay  DelayLength=1  InitialCondition=0  SampleTime=t_simulink
  Flip : DSPFlip
  IC : InitialCondition  Value=ic_sw_So5
  Mux : Mux  Inputs=2
  To Workspace5 : ToWorkspace  VariableName=sw_So5  SampleTime=1/96
  Variable Selector : dspindex/Variable Selector  NumInputs=1  rowsOrCols=Rows  IdxMode=Fixed  Elements=1:(n_sw_inverse-1)  ZerOneIdxMode=One-based  errmode=Clip Index  FillMode=on  FillValues=0
  Out : Outport  VectorParamsAs1DForOutWhenUnconnected=off
  wires:
  IC/1 -> Variable Selector/1
  Delay1/1 -> IC/1
  In/1 -> Mux/1
  Variable Selector/1 -> Mux/2
  Flip/1 -> To Workspace5/1, Out/1
  Mux/1 -> Delay1/1, Flip/1

== system benchmark_ivan_PIANN/SO5_control_paper/Filter_Prediction/DAE_MLP3/Sliding Window/Sliding Window2 ==
  In : Inport
  Delay1 : Delay  DelayLength=1  InitialCondition=0  SampleTime=t_simulink
  Flip : DSPFlip
  IC : InitialCondition  Value=ic_sw_Snh4
  Mux : Mux  Inputs=2
  To Workspace5 : ToWorkspace  VariableName=sw_Q4  SampleTime=1/96
  Variable Selector : dspindex/Variable Selector  NumInputs=1  rowsOrCols=Rows  IdxMode=Fixed  Elements=1:(n_sw_inverse-1)  ZerOneIdxMode=One-based  errmode=Clip Index  FillMode=on  FillValues=0
  Out : Outport  VectorParamsAs1DForOutWhenUnconnected=off
  wires:
  IC/1 -> Variable Selector/1
  Delay1/1 -> IC/1
  In/1 -> Mux/1
  Variable Selector/1 -> Mux/2
  Flip/1 -> To Workspace5/1, Out/1
  Mux/1 -> Delay1/1, Flip/1

== system benchmark_ivan_PIANN/SO5_control_paper/Filter_Prediction/DAE_MLP3/Sliding Window/Sliding Window5 ==
  In : Inport
  Delay1 : Delay  DelayLength=1  InitialCondition=0  SampleTime=t_simulink
  Flip : DSPFlip
  IC : InitialCondition  Value=ic_sw_Sno4
  Mux : Mux  Inputs=2
  To Workspace5 : ToWorkspace  VariableName=sw_TSS4  SampleTime=1/96
  Variable Selector : dspindex/Variable Selector  NumInputs=1  rowsOrCols=Rows  IdxMode=Fixed  Elements=1:(n_sw_inverse-1)  ZerOneIdxMode=One-based  errmode=Clip Index  FillMode=on  FillValues=0
  Out : Outport  VectorParamsAs1DForOutWhenUnconnected=off
  wires:
  IC/1 -> Variable Selector/1
  Delay1/1 -> IC/1
  In/1 -> Mux/1
  Variable Selector/1 -> Mux/2
  Flip/1 -> To Workspace5/1, Out/1
  Mux/1 -> Delay1/1, Flip/1

== system benchmark_ivan_PIANN/SO5_control_paper/Filter_Prediction/DAE_MLP3/Sliding Window/Sliding Window7 ==
  In : Inport
  Delay1 : Delay  DelayLength=1  InitialCondition=0  SampleTime=t_simulink
  Flip : DSPFlip
  IC : InitialCondition  Value=ic_sw_So4
  Mux : Mux  Inputs=2
  To Workspace5 : ToWorkspace  VariableName=sw_Snh4  SampleTime=1/96
  Variable Selector : dspindex/Variable Selector  NumInputs=1  rowsOrCols=Rows  IdxMode=Fixed  Elements=1:(n_sw_inverse-1)  ZerOneIdxMode=One-based  errmode=Clip Index  FillMode=on  FillValues=0
  Out : Outport  VectorParamsAs1DForOutWhenUnconnected=off
  wires:
  IC/1 -> Variable Selector/1
  Delay1/1 -> IC/1
  In/1 -> Mux/1
  Variable Selector/1 -> Mux/2
  Flip/1 -> To Workspace5/1, Out/1
  Mux/1 -> Delay1/1, Flip/1

== system benchmark_ivan_PIANN/SO5_control_paper/Filter_Prediction/DAE_lstm/Data Preprocesing Direct/Normalizer1 ==
  Data Input : Inport
  Normalization Values : MATLAB Function  TreatAsAtomicUnit=on
  Data Normalized : Outport  VectorParamsAs1DForOutWhenUnconnected=off
  wires:
  Normalization Values/1(data_norm) -> Data Normalized/1
  Data Input/1 -> Normalization Values/1(data_input)

== system benchmark_ivan_PIANN/SO5_control_paper/Filter_Prediction/DAE_lstm/Sliding Window/Sliding Window1 ==
  In : Inport
  Delay : Delay  DelayLength=1  InitialCondition=0
  Flip : DSPFlip
  IC : InitialCondition  Value=zeros(8,1)
  Mux : Mux  Inputs=2
  Variable Selector : dspindex/Variable Selector  NumInputs=1  rowsOrCols=Rows  IdxMode=Fixed  Elements=1:7  ZerOneIdxMode=One-based  errmode=Clip Index  FillMode=on  FillValues=0
  Out : Outport  VectorParamsAs1DForOutWhenUnconnected=off
  wires:
  IC/1 -> Variable Selector/1
  Delay/1 -> IC/1
  In/1 -> Mux/1
  Variable Selector/1 -> Mux/2
  Flip/1 -> Out/1
  Mux/1 -> Flip/1, Delay/1

== system benchmark_ivan_PIANN/SO5_control_paper/Filter_Prediction/DAE_lstm/Sliding Window/Sliding Window2 ==
  In : Inport
  Delay : Delay  DelayLength=1  InitialCondition=0
  Flip : DSPFlip
  IC : InitialCondition  Value=zeros(n_sw_inverse,1)
  Mux : Mux  Inputs=2
  Variable Selector : dspindex/Variable Selector  NumInputs=1  rowsOrCols=Rows  IdxMode=Fixed  Elements=1:(n_sw_inverse-1)  ZerOneIdxMode=One-based  errmode=Clip Index  FillMode=on  FillValues=0
  Out : Outport  VectorParamsAs1DForOutWhenUnconnected=off
  wires:
  IC/1 -> Variable Selector/1
  Delay/1 -> IC/1
  In/1 -> Mux/1
  Variable Selector/1 -> Mux/2
  Flip/1 -> Out/1
  Mux/1 -> Delay/1, Flip/1

== system benchmark_ivan_PIANN/SO5_control_paper/Filter_Prediction/DAE_lstm/Sliding Window/Sliding Window3 ==
  In : Inport
  Delay : Delay  DelayLength=1  InitialCondition=0
  Flip : DSPFlip
  IC : InitialCondition  Value=zeros(n_sw_inverse,1)
  Mux : Mux  Inputs=2
  Variable Selector : dspindex/Variable Selector  NumInputs=1  rowsOrCols=Rows  IdxMode=Fixed  Elements=1:(n_sw_inverse-1)  ZerOneIdxMode=One-based  errmode=Clip Index  FillMode=on  FillValues=0
  Out : Outport  VectorParamsAs1DForOutWhenUnconnected=off
  wires:
  IC/1 -> Variable Selector/1
  Delay/1 -> IC/1
  In/1 -> Mux/1
  Variable Selector/1 -> Mux/2
  Flip/1 -> Out/1
  Mux/1 -> Delay/1, Flip/1

== system benchmark_ivan_PIANN/SO5_control_paper/Filter_Prediction/DAE_lstm/Sliding Window/Sliding Window4 ==
  In : Inport
  Delay : Delay  DelayLength=1  InitialCondition=0
  Flip : DSPFlip
  IC : InitialCondition  Value=zeros(n_sw_inverse,1)
  Mux : Mux  Inputs=2
  Variable Selector : dspindex/Variable Selector  NumInputs=1  rowsOrCols=Rows  IdxMode=Fixed  Elements=1:(n_sw_inverse-1)  ZerOneIdxMode=One-based  errmode=Clip Index  FillMode=on  FillValues=0
  Out : Outport  VectorParamsAs1DForOutWhenUnconnected=off
  wires:
  IC/1 -> Variable Selector/1
  Delay/1 -> IC/1
  In/1 -> Mux/1
  Variable Selector/1 -> Mux/2
  Flip/1 -> Out/1
  Mux/1 -> Delay/1, Flip/1

== system benchmark_ivan_PIANN/SO5_control_paper/Filter_Prediction/DAE_lstm/Sliding Window/Sliding Window6 ==
  In : Inport
  Delay : Delay  DelayLength=1  InitialCondition=0
  Flip : DSPFlip
  IC : InitialCondition  Value=zeros(n_sw_inverse,1)
  Mux : Mux  Inputs=2
  Variable Selector : dspindex/Variable Selector  NumInputs=1  rowsOrCols=Rows  IdxMode=Fixed  Elements=1:(n_sw_inverse-1)  ZerOneIdxMode=One-based  errmode=Clip Index  FillMode=on  FillValues=0
  Out : Outport  VectorParamsAs1DForOutWhenUnconnected=off
  wires:
  IC/1 -> Variable Selector/1
  Delay/1 -> IC/1
  In/1 -> Mux/1
  Variable Selector/1 -> Mux/2
  Flip/1 -> Out/1
  Mux/1 -> Delay/1, Flip/1

== system benchmark_ivan_PIANN/SO5_control_paper/Filter_Prediction/Direct Prediction LSTM4/Sliding Window 1/Sliding Window Buffer ==
  In1 : Inport
  Buffer1 : Buffer  N=n_sw  V=n_sw-1  ic=145
  Reshape : Reshape
  To Workspace5 : ToWorkspace  VariableName=sw_Kla1  SampleTime=-1
  Zero-Order Hold : ZeroOrderHold  SampleTime=-1
  Out1 : Outport
  wires:
  Buffer1/1 -> Reshape/1
  Reshape/1 -> To Workspace5/1, Out1/1
  In1/1 -> Zero-Order Hold/1
  Zero-Order Hold/1 -> Buffer1/1

== system benchmark_ivan_PIANN/SO5_control_paper/Filter_Prediction/Direct Prediction LSTM4/Sliding Window 1/Sliding Window2 ==
  In : Inport
  Delay1 : Delay  DelayLength=1  InitialCondition=145
  Flip : DSPFlip
  IC : InitialCondition  Value=ic_sw_Kla
  Mux : Mux  Inputs=2
  To Workspace5 : ToWorkspace  VariableName=sw_Kla  SampleTime=-1
  Variable Selector : dspindex/Variable Selector  NumInputs=1  rowsOrCols=Rows  IdxMode=Fixed  Elements=1:(n_sw_inverse-1)  ZerOneIdxMode=One-based  errmode=Clip Index  FillMode=on  FillValues=0
  Out : Outport  VectorParamsAs1DForOutWhenUnconnected=off
  wires:
  IC/1 -> Variable Selector/1
  Delay1/1 -> IC/1
  In/1 -> Mux/1
  Variable Selector/1 -> Mux/2
  Flip/1 -> To Workspace5/1, Out/1
  Mux/1 -> Delay1/1, Flip/1

== system benchmark_ivan_PIANN/SO5_control_paper/Filter_Prediction/Direct Prediction LSTM4/Sliding Window 48 /Sliding Window1 ==
  In : Inport
  Delay : Delay  DelayLength=1  InitialCondition=0
  Flip : DSPFlip
  IC : InitialCondition  Value=zeros(8,1)
  Mux : Mux  Inputs=2
  Variable Selector : dspindex/Variable Selector  NumInputs=1  rowsOrCols=Rows  IdxMode=Fixed  Elements=1:7  ZerOneIdxMode=One-based  errmode=Clip Index  FillMode=on  FillValues=0
  Out : Outport  VectorParamsAs1DForOutWhenUnconnected=off
  wires:
  IC/1 -> Variable Selector/1
  Delay/1 -> IC/1
  In/1 -> Mux/1
  Variable Selector/1 -> Mux/2
  Flip/1 -> Out/1
  Mux/1 -> Flip/1, Delay/1

== system benchmark_ivan_PIANN/SO5_control_paper/Filter_Prediction/Direct Prediction LSTM4/Sliding Window 48 /Sliding Window2 ==
  In : Inport
  Delay1 : Delay  DelayLength=1  InitialCondition=0  SampleTime=t_simulink
  Flip : DSPFlip
  IC : InitialCondition  Value=ic_sw_Kla
  Mux : Mux  Inputs=2
  To Workspace5 : ToWorkspace  VariableName=sw_Kla  SampleTime=1/96
  Variable Selector : dspindex/Variable Selector  NumInputs=1  rowsOrCols=Rows  IdxMode=Fixed  Elements=1:(n_sw_inverse-1)  ZerOneIdxMode=One-based  errmode=Clip Index  FillMode=on  FillValues=0
  Out : Outport  VectorParamsAs1DForOutWhenUnconnected=off
  wires:
  IC/1 -> Variable Selector/1
  Delay1/1 -> IC/1
  In/1 -> Mux/1
  Variable Selector/1 -> Mux/2
  Flip/1 -> To Workspace5/1, Out/1
  Mux/1 -> Delay1/1, Flip/1

== system benchmark_ivan_PIANN/SO5_control_paper/Filter_Prediction/Direct Prediction LSTM4/Sliding Window 64/Sliding Window1 ==
  In : Inport
  Delay : Delay  DelayLength=1  InitialCondition=0
  Flip : DSPFlip
  IC : InitialCondition  Value=zeros(8,1)
  Mux : Mux  Inputs=2
  Variable Selector : dspindex/Variable Selector  NumInputs=1  rowsOrCols=Rows  IdxMode=Fixed  Elements=1:7  ZerOneIdxMode=One-based  errmode=Clip Index  FillMode=on  FillValues=0
  Out : Outport  VectorParamsAs1DForOutWhenUnconnected=off
  wires:
  IC/1 -> Variable Selector/1
  Delay/1 -> IC/1
  In/1 -> Mux/1
  Variable Selector/1 -> Mux/2
  Flip/1 -> Out/1
  Mux/1 -> Flip/1, Delay/1

== system benchmark_ivan_PIANN/SO5_control_paper/Filter_Prediction/Direct Prediction LSTM4/Sliding Window 64/Sliding Window2 ==
  In : Inport
  Delay1 : Delay  DelayLength=1  InitialCondition=0  SampleTime=t_simulink
  Flip : DSPFlip
  IC : InitialCondition  Value=ic_sw_Kla
  Mux : Mux  Inputs=2
  To Workspace5 : ToWorkspace  VariableName=sw_Kla  SampleTime=1/96
  Variable Selector : dspindex/Variable Selector  NumInputs=1  rowsOrCols=Rows  IdxMode=Fixed  Elements=1:(n_sw_inverse-1)  ZerOneIdxMode=One-based  errmode=Clip Index  FillMode=on  FillValues=0
  Out : Outport  VectorParamsAs1DForOutWhenUnconnected=off
  wires:
  IC/1 -> Variable Selector/1
  Delay1/1 -> IC/1
  In/1 -> Mux/1
  Variable Selector/1 -> Mux/2
  Flip/1 -> To Workspace5/1, Out/1
  Mux/1 -> Delay1/1, Flip/1

== system benchmark_ivan_PIANN/SO5_control_paper/Filter_Prediction/Direct Prediction LSTM4/Sliding Window 64 with So5/Sliding Window1 ==
  In : Inport
  Delay : Delay  DelayLength=1  InitialCondition=0
  Flip : DSPFlip
  IC : InitialCondition  Value=zeros(8,1)
  Mux : Mux  Inputs=2
  Variable Selector : dspindex/Variable Selector  NumInputs=1  rowsOrCols=Rows  IdxMode=Fixed  Elements=1:7  ZerOneIdxMode=One-based  errmode=Clip Index  FillMode=on  FillValues=0
  Out : Outport  VectorParamsAs1DForOutWhenUnconnected=off
  wires:
  IC/1 -> Variable Selector/1
  Delay/1 -> IC/1
  In/1 -> Mux/1
  Variable Selector/1 -> Mux/2
  Flip/1 -> Out/1
  Mux/1 -> Flip/1, Delay/1

== system benchmark_ivan_PIANN/SO5_control_paper/Filter_Prediction/Direct Prediction LSTM4/Sliding Window 64 with So5/Sliding Window2 ==
  In : Inport
  Delay1 : Delay  DelayLength=1  InitialCondition=0  SampleTime=t_simulink
  Flip : DSPFlip
  IC : InitialCondition  Value=ic_sw_Kla
  Mux : Mux  Inputs=2
  To Workspace5 : ToWorkspace  VariableName=sw_Kla  SampleTime=1/96
  Variable Selector : dspindex/Variable Selector  NumInputs=1  rowsOrCols=Rows  IdxMode=Fixed  Elements=1:(n_sw_inverse-1)  ZerOneIdxMode=One-based  errmode=Clip Index  FillMode=on  FillValues=0
  Out : Outport  VectorParamsAs1DForOutWhenUnconnected=off
  wires:
  IC/1 -> Variable Selector/1
  Delay1/1 -> IC/1
  In/1 -> Mux/1
  Variable Selector/1 -> Mux/2
  Flip/1 -> To Workspace5/1, Out/1
  Mux/1 -> Delay1/1, Flip/1

== matlab function benchmark_ivan_PIANN/SO5_control_paper/Filter_Prediction/DAE_MLP2/Data Preprocessing Direct1/Denormalization Values ==
  data: mean_scaler_dae_out parameter; data_dir output; std_scaler_dae_out parameter; data_input input
function data_dir = descaler(mean_scaler_dae_out, std_scaler_dae_out, data_input)
%#codegen
data_dir = zeros(1, 64);

mean_output_3 = mean_scaler_dae_out';
std_output_3 = std_scaler_dae_out';

data_dir = std_output_3.*data_input + mean_output_3;
